simulink model "Last_Model_Interior_team"  (R2017b)
settings: Solver=VariableStepAuto  SolverName=FixedStepDiscrete  StartTime=0.0  StopTime=10  FixedStep=1e-6
PreLoadFcn:
  | %% Motor Parameters
  | Rs=6.9*10^-3;
  | Ld=220*10^-6;
  | Lq=265.4*10^-6;
  | Pm=87.78*10^-3;
  | P=4;
  | b=0.0019;
  | J=0.13;
  | f=50;
  | P_Rated=100000;
  | N_Rated=6320;
  | N_max=30000;
  | Tfl=P_Rated/(N_Rated*(2*pi/60));
  | Tl=0;
  | 
  | %% hardware impl
  | Vdc=340;
  | clocking=100;
  | fs=10000;
  | Ts=1/fs;
  | Irated=500;
  | Imax=500;
  | Id_MAX=-(Pm/Ld);
  | I_Limit=Irated;
  | I_fw=I_Limit;
  | Vmax=Vdc/sqrt(3);
  | update=2;
  | 
  | 
  | %% Inverter
  | Vdc=340;
  | deadtime=1e-6;
  | 
  | 
  | 
  | %% Tuning OF Id_Pole_Placment
  | zeta_Id=0.707;
  | Gamma_Id=0.9;
  | Wn_Id=(1/(1-Gamma_Id))*(Rs/Ld);
  | Kc_Id=(2*zeta_Id*Ld*Wn_Id)-Rs;
  | TAW_Id=((2*zeta_Id*Wn_Id*Ld)-Rs)/(Ld*Wn_Id*Wn_Id);
  | 
  | %% Tuning OF Iq_Pole_Placment
  | zeta_Iq=0.707;
  | Gamma_Iq=0.9;
  | Wn_Iq=(1/(1-Gamma_Iq))*(Rs/Lq);
  | Kc_Iq=(2*zeta_Iq*Lq*Wn_Iq)-Rs;
  | TAW_Iq=((2*zeta_Iq*Wn_Iq*Lq)-Rs)/(Lq*Wn_Iq*Wn_Iq);
  | 
  | 
  | 
  | %% Tuning of PI Using Symmetric Optimum For q phase
  | Tc=(1/fs)/update;
  | A=8;
  | Kp_SO_q=Lq/(A*(Tc)*1.5);
  | Ki_SO_q=1/((A^2)*1.5*Tc);
  | %% Tuning of PI Using Symmetric Optimum For d phase
  | Kp_SO_d=Ld/(A*(Tc)*1.5);
  | Ki_SO_d=1/((A^2)*1.5*Tc);
  | 
  | ... (+20 lines)
InitFcn:
  | %% Motor Parameters
  | Rs=6.9*10^-3;
  | Ld=220*10^-6;
  | Lq=265.4*10^-6;
  | Pm=87.78*10^-3;
  | P=4;
  | b=0.0019;
  | J=0.13;
  | f=50;
  | P_Rated=100000;
  | N_Rated=6320;
  | N_max=30000;
  | Tfl=P_Rated/(N_Rated*(2*pi/60));
  | Tl=0;
  | 
  | %% hardware impl
  | Vdc=340;
  | clocking=100;
  | fs=10000;
  | Ts=1/fs;
  | Irated=500;
  | Imax=500;
  | Id_MAX=-(Pm/Ld);
  | I_Limit=Irated;
  | I_fw=I_Limit;
  | Vmax=Vdc/sqrt(3);
  | update=2;
  | 
  | %% Inverter
  | Vdc=340;
  | deadtime=1e-6;
  | 
  | 
  | 
  | %% Tuning OF Id_Pole_Placment
  | zeta_Id=0.707;
  | Gamma_Id=0.9;
  | Wn_Id=(1/(1-Gamma_Id))*(Rs/Ld);
  | Kc_Id=(2*zeta_Id*Ld*Wn_Id)-Rs;
  | TAW_Id=((2*zeta_Id*Wn_Id*Ld)-Rs)/(Ld*Wn_Id*Wn_Id);
  | 
  | %% Tuning OF Iq_Pole_Placment
  | zeta_Iq=0.707;
  | Gamma_Iq=0.9;
  | Wn_Iq=(1/(1-Gamma_Iq))*(Rs/Lq);
  | Kc_Iq=(2*zeta_Iq*Lq*Wn_Iq)-Rs;
  | TAW_Iq=((2*zeta_Iq*Wn_Iq*Lq)-Rs)/(Lq*Wn_Iq*Wn_Iq);
  | 
  | 
  | 
  | %% Tuning of PI Using Symmetric Optimum For q phase
  | Tc=(1/fs)/update;
  | A=8;
  | Kp_SO_q=Lq/(A*(Tc)*1.5);
  | Ki_SO_q=1/((A^2)*1.5*Tc);
  | %% Tuning of PI Using Symmetric Optimum For d phase
  | Kp_SO_d=Ld/(A*(Tc)*1.5);
  | Ki_SO_d=1/((A^2)*1.5*Tc);
  | 
  | 
  | ... (+19 lines)
undefined symbols (not defined in the file): DiscIntNeverNeededParam, magnitude
libraries: simulink x81, powerlib x14
(part 2 of 4)

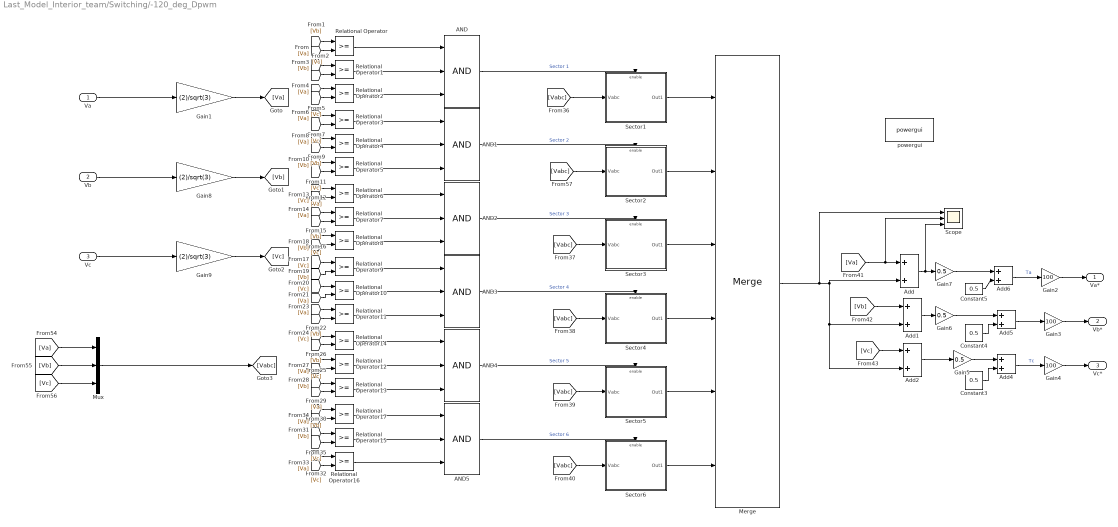
== system Last_Model_Interior_team/Switching/-120_deg_Dpwm ==
  Va : Inport
  Vb : Inport  Port=2
  Vc : Inport  Port=3
  AND{,1..5} (6 alike) : Logic  Inputs=3  IconShape=distinctive  AllPortsSameDT=off  OutDataTypeStr=boolean
  Add{,1..2,4..6} (6 alike) : Sum
  Constant3 : Constant  Value=0.5
  Constant4 : Constant  Value=0.5
  Constant5 : Constant  Value=0.5
  Gain1 : Gain  Gain=(2)/sqrt(3)  RndMeth=Simplest  OutDataTypeStr=Inherit: Same as input  ParamDataTypeStr=Inherit: Same as input
  Gain2 : Gain  Gain=100
  Gain3 : Gain  Gain=100
  Gain4 : Gain  Gain=100
  Gain5 : Gain  Gain=0.5
  Gain6 : Gain  Gain=0.5
  Gain7 : Gain  Gain=0.5
  Gain8 : Gain  Gain=(2)/sqrt(3)  RndMeth=Simplest  OutDataTypeStr=Inherit: Same as input  ParamDataTypeStr=Inherit: Same as input
  Gain9 : Gain  Gain=(2)/sqrt(3)  RndMeth=Simplest  OutDataTypeStr=Inherit: Same as input  ParamDataTypeStr=Inherit: Same as input
  Merge : Merge  Inputs=6
  Mux : Mux  Inputs=3
  Relational Operator{,1..17} (18 alike) : RelationalOperator  OutDataTypeStr=boolean  RndMeth=Simplest
  Scope : Scope  NumInputPorts=3
  Sector1 : Subsystem  TreatAsAtomicUnit=on
  Sector2 : Subsystem  TreatAsAtomicUnit=on
  Sector3 : Subsystem  TreatAsAtomicUnit=on
  Sector4 : Subsystem  TreatAsAtomicUnit=on
  Sector5 : Subsystem  TreatAsAtomicUnit=on
  Sector6 : Subsystem  TreatAsAtomicUnit=on
  powergui : powerlib/powergui  Priority=1  SimulationMode=Discrete  SampleTime=1e-6  frequency=60  Iterations=50  frequencyindice=0  Pbase=100e6  ErrMax=1e-4  UnitsV=kV  UnitsW=MW  buscounter=0  FunctionMessages=off  echomessages=off  EnableUseOfTLC=off  CurrentSourceSwitches=off  DisableSnubberDevices=off  DisableRonSwitches=off  DisableVfSwitches=off  DisplayEquations=off  AutomaticDiscreteSolvers=off  SolverType=Tustin/Backward Euler (TBE)  Interpol=off  ExternalGateDelay=off  methode=off  Ts=100  x0status=blocks  SPID=on  SwTol=0  HookPort=off  NonlinearTolerance=1e-4  nMaxIteration=100  ContinueOnMaxIteration=off  RestoreLinks=warning  ResistiveCurrentMeasurement=off  Frange=[0:2:500]  Ylog=off  Xlog=on  ShowGrid=off  save=off  variable=ZData  structure=0  ZoomFFT=off  StartTime=0.0  cycles=1  DisplayStyle=1  fundamental=60  FreqAxis=off  MaxFrequency=1000  frequencyindicesteady=1  RmsSteady=1  display=off
  Va* : Outport
  Vb* : Outport  Port=2
  Vc* : Outport  Port=3
  wires:
  AND5/1 -> Sector6/Enable  "Sector 6"
  AND4/1 -> Sector5/Enable  "Sector 5"
  AND3/1 -> Sector4/Enable  "Sector 4"
  AND2/1 -> Sector3/Enable  "Sector 3"
  AND1/1 -> Sector2/Enable  "Sector 2"
  AND/1 -> Sector1/Enable  "Sector 1"
  [Va] -> Relational Operator4/1
  [Va] -> Relational Operator2/1
  [Vb] -> Relational Operator11/2
  Relational Operator17/1 -> AND5/1
  [Va] -> Relational Operator12/2
  [Vabc] -> Sector4/1(Vabc)
  [Va] -> Relational Operator16/2
  [Vb] -> Relational Operator13/1
  [Vc] -> Relational Operator5/2
  [Vb] -> Relational Operator/1
  [Vabc] -> Sector5/1(Vabc)
  [Va] -> Scope/2, Add/1
  Relational Operator11/1 -> AND3/3
  [Vb] -> Relational Operator15/1
  [Vc] -> Relational Operator2/2
  Relational Operator16/1 -> AND5/3
  [Va] -> Relational Operator17/2
  Relational Operator15/1 -> AND5/2
  Relational Operator12/1 -> AND4/2
  [Va] -> Relational Operator3/1
  [Va] -> Relational Operator/2
  Relational Operator/1 -> AND/1
  Relational Operator3/1 -> AND1/1
  [Vc] -> Mux/3
  Sector1/1(Out1) -> Merge/1
  Gain4/1 -> Vc*/1
  [Vb] -> Relational Operator1/1
  [Vb] -> Relational Operator4/2
  Gain6/1 -> Add5/1
  [Vb] -> Relational Operator17/1
  Gain2/1 -> Va*/1
  Relational Operator1/1 -> AND/2
  Relational Operator9/1 -> AND3/1
  [Va] -> Relational Operator11/1
  [Va] -> Mux/1
  [Vc] -> Relational Operator12/1
  Relational Operator7/1 -> AND2/2
  [Vabc] -> Sector6/1(Vabc)
  [Vc] -> Relational Operator15/2
  Relational Operator2/1 -> AND/3
  [Vc] -> Relational Operator3/2
  [Vb] -> Mux/2
  [Vc] -> Relational Operator14/1
  [Vc] -> Relational Operator10/1
  Relational Operator13/1 -> AND4/3
  Relational Operator14/1 -> AND4/1
  [Vc] -> Relational Operator9/1
  [Vabc] -> Sector1/1(Vabc)
  Relational Operator10/1 -> AND3/2
  Add1/1 -> Gain6/1
  [Vb] -> Relational Operator5/1
  Relational Operator5/1 -> AND1/3
  Relational Operator4/1 -> AND1/2
  Relational Operator6/1 -> AND2/1
  Relational Operator8/1 -> AND2/3
  [Vc] -> Relational Operator1/2
  [Vc] -> Relational Operator8/1
  [Vabc] -> Sector2/1(Vabc)
  [Vc] -> Relational Operator16/1
  [Vb] -> Relational Operator14/2
  [Vb] -> Relational Operator9/2
  [Vb] -> Relational Operator7/2
  [Vc] -> Relational Operator6/2
  [Va] -> Relational Operator6/1
  Gain3/1 -> Vb*/1
  [Va] -> Relational Operator7/1
  [Va] -> Relational Operator13/2
  [Vb] -> Relational Operator8/2
  [Va] -> Relational Operator10/2
  Sector2/1(Out1) -> Merge/2
  Sector6/1(Out1) -> Merge/6
  [Vabc] -> Sector3/1(Vabc)
  Sector3/1(Out1) -> Merge/3
  Sector5/1(Out1) -> Merge/5
  Sector4/1(Out1) -> Merge/4
  [Vc] -> Add2/1
  [Vb] -> Add1/1
  Gain5/1 -> Add4/1
  Constant3/1 -> Add4/2
  Constant4/1 -> Add5/2
  Gain7/1 -> Add6/1
  Constant5/1 -> Add6/2
  Add2/1 -> Gain5/1
  Add5/1 -> Gain3/1
  Add4/1 -> Gain4/1  "Tc"
  Add6/1 -> Gain2/1  "Ta"
  Mux/1 -> [Vabc]
  Vc/1 -> Gain9/1
  Vb/1 -> Gain8/1
  Va/1 -> Gain1/1
  Merge/1 -> Scope/1, Add/2, Add2/2, Add1/2
  Add/1 -> Scope/3, Gain7/1
  Gain1/1 -> [Va]
  Gain8/1 -> [Vb]
  Gain9/1 -> [Vc]

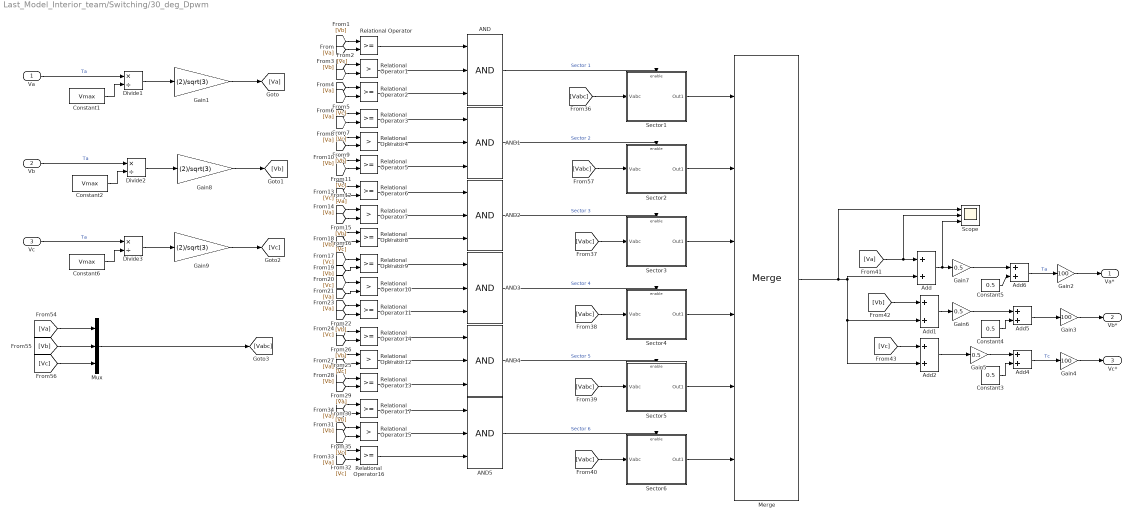
== system Last_Model_Interior_team/Switching/30_deg_Dpwm ==
  Va : Inport
  Vb : Inport  Port=2
  Vc : Inport  Port=3
  AND{,1..5} (6 alike) : Logic  Inputs=3  IconShape=distinctive  AllPortsSameDT=off  OutDataTypeStr=boolean
  Add{,1..2,4..6} (6 alike) : Sum
  Constant1 : Constant  Value=Vmax
  Constant2 : Constant  Value=Vmax
  Constant3 : Constant  Value=0.5
  Constant4 : Constant  Value=0.5
  Constant5 : Constant  Value=0.5
  Constant6 : Constant  Value=Vmax
  Divide1 : Product  Inputs=*/
  Divide2 : Product  Inputs=*/
  Divide3 : Product  Inputs=*/
  Gain1 : Gain  Gain=(2)/sqrt(3)  RndMeth=Simplest  OutDataTypeStr=Inherit: Same as input  ParamDataTypeStr=Inherit: Same as input
  Gain2 : Gain  Gain=100
  Gain3 : Gain  Gain=100
  Gain4 : Gain  Gain=100
  Gain5 : Gain  Gain=0.5
  Gain6 : Gain  Gain=0.5
  Gain7 : Gain  Gain=0.5
  Gain8 : Gain  Gain=(2)/sqrt(3)  RndMeth=Simplest  OutDataTypeStr=Inherit: Same as input  ParamDataTypeStr=Inherit: Same as input
  Gain9 : Gain  Gain=(2)/sqrt(3)  RndMeth=Simplest  OutDataTypeStr=Inherit: Same as input  ParamDataTypeStr=Inherit: Same as input
  Merge : Merge  Inputs=6
  Mux : Mux  Inputs=3
  Relational Operator{,2..3,5..6,8..9,11,13..14,16..17} (12 alike) : RelationalOperator  OutDataTypeStr=boolean  RndMeth=Simplest
  Relational Operator{1,4,7,10,12,15} (6 alike) : RelationalOperator  Operator=>  OutDataTypeStr=boolean  RndMeth=Simplest
  Scope : Scope  NumInputPorts=3
  Sector1 : Subsystem  TreatAsAtomicUnit=on
  Sector2 : Subsystem  TreatAsAtomicUnit=on
  Sector3 : Subsystem  TreatAsAtomicUnit=on
  Sector4 : Subsystem  TreatAsAtomicUnit=on
  Sector5 : Subsystem  TreatAsAtomicUnit=on
  Sector6 : Subsystem  TreatAsAtomicUnit=on
  Va* : Outport
  Vb* : Outport  Port=2
  Vc* : Outport  Port=3
  wires:
  Add/1 -> Gain7/1, Scope/3
  Merge/1 -> Add1/2, Add2/2, Add/2, Scope/1
  Add6/1 -> Gain2/1  "Ta"
  Add4/1 -> Gain4/1  "Tc"
  Add5/1 -> Gain3/1
  Add2/1 -> Gain5/1
  Constant5/1 -> Add6/2
  Gain7/1 -> Add6/1
  Constant4/1 -> Add5/2
  Constant3/1 -> Add4/2
  Gain5/1 -> Add4/1
  [Vb] -> Add1/1
  [Vc] -> Add2/1
  Sector4/1(Out1) -> Merge/4
  Sector5/1(Out1) -> Merge/5
  Sector3/1(Out1) -> Merge/3
  [Vabc] -> Sector3/1(Vabc)
  Sector6/1(Out1) -> Merge/6
  Sector2/1(Out1) -> Merge/2
  [Va] -> Relational Operator10/2
  [Vb] -> Relational Operator8/2
  [Va] -> Relational Operator13/2
  [Va] -> Relational Operator7/1
  Gain3/1 -> Vb*/1
  [Va] -> Relational Operator6/1
  [Vc] -> Relational Operator6/2
  [Vb] -> Relational Operator7/2
  [Vb] -> Relational Operator9/2
  [Vb] -> Relational Operator14/2
  [Vc] -> Relational Operator16/1
  [Vabc] -> Sector2/1(Vabc)
  [Vc] -> Relational Operator8/1
  [Vc] -> Relational Operator1/2
  Relational Operator8/1 -> AND2/3
  Relational Operator6/1 -> AND2/1
  Relational Operator4/1 -> AND1/2
  Relational Operator5/1 -> AND1/3
  [Vb] -> Relational Operator5/1
  Add1/1 -> Gain6/1
  Relational Operator10/1 -> AND3/2
  [Vabc] -> Sector1/1(Vabc)
  [Vc] -> Relational Operator9/1
  Relational Operator14/1 -> AND4/1
  Relational Operator13/1 -> AND4/3
  [Vc] -> Relational Operator10/1
  [Vc] -> Relational Operator14/1
  [Vc] -> Relational Operator3/2
  Relational Operator2/1 -> AND/3
  [Vc] -> Relational Operator15/2
  [Vabc] -> Sector6/1(Vabc)
  Relational Operator7/1 -> AND2/2
  [Vc] -> Relational Operator12/1
  [Va] -> Relational Operator11/1
  Relational Operator9/1 -> AND3/1
  Relational Operator1/1 -> AND/2
  Gain2/1 -> Va*/1
  [Vb] -> Relational Operator17/1
  Gain6/1 -> Add5/1
  [Vb] -> Relational Operator4/2
  [Vb] -> Relational Operator1/1
  Gain4/1 -> Vc*/1
  Sector1/1(Out1) -> Merge/1
  Relational Operator3/1 -> AND1/1
  Relational Operator/1 -> AND/1
  [Va] -> Relational Operator/2
  [Va] -> Relational Operator3/1
  Relational Operator12/1 -> AND4/2
  Relational Operator15/1 -> AND5/2
  [Va] -> Relational Operator17/2
  Relational Operator16/1 -> AND5/3
  [Vc] -> Relational Operator2/2
  [Vb] -> Relational Operator15/1
  Relational Operator11/1 -> AND3/3
  [Va] -> Add/1, Scope/2
  [Vabc] -> Sector5/1(Vabc)
  [Vb] -> Relational Operator/1
  [Vc] -> Relational Operator5/2
  [Vb] -> Relational Operator13/1
  [Va] -> Relational Operator16/2
  [Vabc] -> Sector4/1(Vabc)
  [Va] -> Relational Operator12/2
  Relational Operator17/1 -> AND5/1
  [Vb] -> Relational Operator11/2
  [Va] -> Relational Operator2/1
  [Va] -> Relational Operator4/1
  AND/1 -> Sector1/Enable  "Sector 1"
  AND1/1 -> Sector2/Enable  "Sector 2"
  AND2/1 -> Sector3/Enable  "Sector 3"
  AND3/1 -> Sector4/Enable  "Sector 4"
  AND4/1 -> Sector5/Enable  "Sector 5"
  AND5/1 -> Sector6/Enable  "Sector 6"
  Constant1/1 -> Divide1/2
  Vb/1 -> Divide2/1  "Ta"
  Divide1/1 -> Gain1/1
  Constant6/1 -> Divide3/2
  Divide3/1 -> Gain9/1
  Vc/1 -> Divide3/1  "Ta"
  Constant2/1 -> Divide2/2
  Divide2/1 -> Gain8/1
  Mux/1 -> [Vabc]
  [Vb] -> Mux/2
  Gain1/1 -> [Va]
  [Vc] -> Mux/3
  [Va] -> Mux/1
  Gain8/1 -> [Vb]
  Gain9/1 -> [Vc]
  Va/1 -> Divide1/1  "Ta"

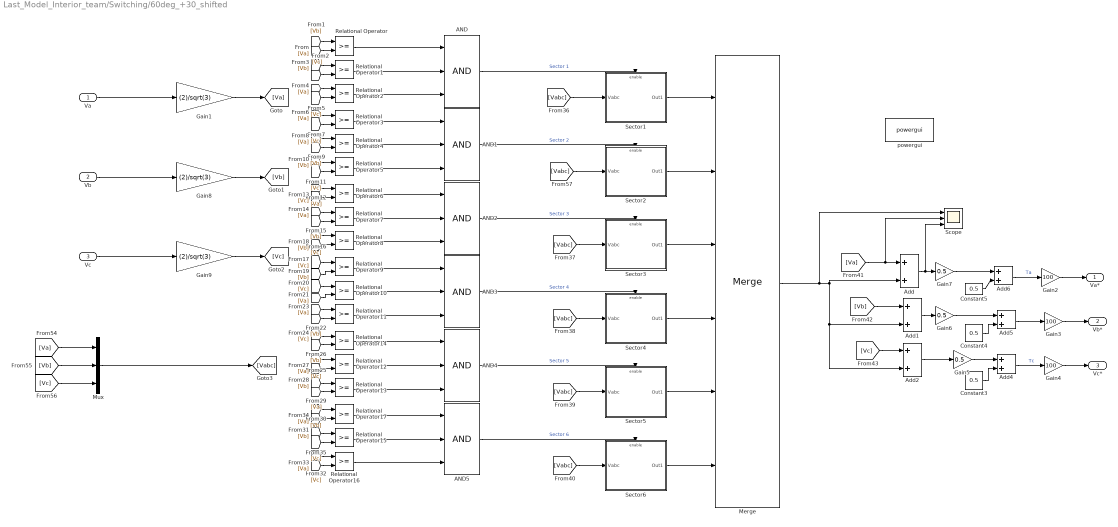
== system Last_Model_Interior_team/Switching/60deg_+30_shifted ==
  Va : Inport
  Vb : Inport  Port=2
  Vc : Inport  Port=3
  AND{,1..5} (6 alike) : Logic  Inputs=3  IconShape=distinctive  AllPortsSameDT=off  OutDataTypeStr=boolean
  Add{,1..2,4..6} (6 alike) : Sum
  Constant3 : Constant  Value=0.5
  Constant4 : Constant  Value=0.5
  Constant5 : Constant  Value=0.5
  Gain1 : Gain  Gain=(2)/sqrt(3)  RndMeth=Simplest  OutDataTypeStr=Inherit: Same as input  ParamDataTypeStr=Inherit: Same as input
  Gain2 : Gain  Gain=100
  Gain3 : Gain  Gain=100
  Gain4 : Gain  Gain=100
  Gain5 : Gain  Gain=0.5
  Gain6 : Gain  Gain=0.5
  Gain7 : Gain  Gain=0.5
  Gain8 : Gain  Gain=(2)/sqrt(3)  RndMeth=Simplest  OutDataTypeStr=Inherit: Same as input  ParamDataTypeStr=Inherit: Same as input
  Gain9 : Gain  Gain=(2)/sqrt(3)  RndMeth=Simplest  OutDataTypeStr=Inherit: Same as input  ParamDataTypeStr=Inherit: Same as input
  Merge : Merge  Inputs=6
  Mux : Mux  Inputs=3
  Relational Operator{,1..17} (18 alike) : RelationalOperator  OutDataTypeStr=boolean  RndMeth=Simplest
  Scope : Scope  NumInputPorts=3
  Sector1 : Subsystem  TreatAsAtomicUnit=on
  Sector2 : Subsystem  TreatAsAtomicUnit=on
  Sector3 : Subsystem  TreatAsAtomicUnit=on
  Sector4 : Subsystem  TreatAsAtomicUnit=on
  Sector5 : Subsystem  TreatAsAtomicUnit=on
  Sector6 : Subsystem  TreatAsAtomicUnit=on
  powergui : powerlib/powergui  Priority=1  SimulationMode=Discrete  SampleTime=1e-6  frequency=60  Iterations=50  frequencyindice=0  Pbase=100e6  ErrMax=1e-4  UnitsV=kV  UnitsW=MW  buscounter=0  FunctionMessages=off  echomessages=off  EnableUseOfTLC=off  CurrentSourceSwitches=off  DisableSnubberDevices=off  DisableRonSwitches=off  DisableVfSwitches=off  DisplayEquations=off  AutomaticDiscreteSolvers=off  SolverType=Tustin/Backward Euler (TBE)  Interpol=off  ExternalGateDelay=off  methode=off  Ts=100  x0status=blocks  SPID=on  SwTol=0  HookPort=off  NonlinearTolerance=1e-4  nMaxIteration=100  ContinueOnMaxIteration=off  RestoreLinks=warning  ResistiveCurrentMeasurement=off  Frange=[0:2:500]  Ylog=off  Xlog=on  ShowGrid=off  save=off  variable=ZData  structure=0  ZoomFFT=off  StartTime=0.0  cycles=1  DisplayStyle=1  fundamental=60  FreqAxis=off  MaxFrequency=1000  frequencyindicesteady=1  RmsSteady=1  display=off
  Va* : Outport
  Vb* : Outport  Port=2
  Vc* : Outport  Port=3
  wires:
  [Va] -> Relational Operator4/1
  [Va] -> Relational Operator2/1
  [Vb] -> Relational Operator11/2
  AND5/1 -> Sector6/Enable  "Sector 6"
  Relational Operator17/1 -> AND5/1
  [Va] -> Relational Operator12/2
  [Vabc] -> Sector4/1(Vabc)
  [Va] -> Relational Operator16/2
  AND3/1 -> Sector4/Enable  "Sector 4"
  AND/1 -> Sector1/Enable  "Sector 1"
  [Vb] -> Relational Operator13/1
  [Vc] -> Relational Operator5/2
  [Vb] -> Relational Operator/1
  [Vabc] -> Sector5/1(Vabc)
  [Va] -> Scope/2, Add/1
  Relational Operator11/1 -> AND3/3
  [Vb] -> Relational Operator15/1
  [Vc] -> Relational Operator2/2
  Relational Operator16/1 -> AND5/3
  [Va] -> Relational Operator17/2
  Relational Operator15/1 -> AND5/2
  Relational Operator12/1 -> AND4/2
  [Va] -> Relational Operator3/1
  [Va] -> Relational Operator/2
  Relational Operator/1 -> AND/1
  AND4/1 -> Sector5/Enable  "Sector 5"
  Relational Operator3/1 -> AND1/1
  [Vc] -> Mux/3
  Sector1/1(Out1) -> Merge/1
  Gain4/1 -> Vc*/1
  [Vb] -> Relational Operator1/1
  [Vb] -> Relational Operator4/2
  Gain6/1 -> Add5/1
  [Vb] -> Relational Operator17/1
  Gain2/1 -> Va*/1
  Relational Operator1/1 -> AND/2
  Relational Operator9/1 -> AND3/1
  [Va] -> Relational Operator11/1
  [Va] -> Mux/1
  [Vc] -> Relational Operator12/1
  AND2/1 -> Sector3/Enable  "Sector 3"
  Relational Operator7/1 -> AND2/2
  [Vabc] -> Sector6/1(Vabc)
  [Vc] -> Relational Operator15/2
  Relational Operator2/1 -> AND/3
  [Vc] -> Relational Operator3/2
  [Vb] -> Mux/2
  [Vc] -> Relational Operator14/1
  [Vc] -> Relational Operator10/1
  Relational Operator13/1 -> AND4/3
  Relational Operator14/1 -> AND4/1
  [Vc] -> Relational Operator9/1
  [Vabc] -> Sector1/1(Vabc)
  Relational Operator10/1 -> AND3/2
  Add1/1 -> Gain6/1
  [Vb] -> Relational Operator5/1
  Relational Operator5/1 -> AND1/3
  Relational Operator4/1 -> AND1/2
  Relational Operator6/1 -> AND2/1
  Relational Operator8/1 -> AND2/3
  [Vc] -> Relational Operator1/2
  [Vc] -> Relational Operator8/1
  [Vabc] -> Sector2/1(Vabc)
  [Vc] -> Relational Operator16/1
  [Vb] -> Relational Operator14/2
  [Vb] -> Relational Operator9/2
  [Vb] -> Relational Operator7/2
  [Vc] -> Relational Operator6/2
  [Va] -> Relational Operator6/1
  Gain3/1 -> Vb*/1
  [Va] -> Relational Operator7/1
  [Va] -> Relational Operator13/2
  [Vb] -> Relational Operator8/2
  [Va] -> Relational Operator10/2
  Sector2/1(Out1) -> Merge/2
  Sector6/1(Out1) -> Merge/6
  [Vabc] -> Sector3/1(Vabc)
  Sector3/1(Out1) -> Merge/3
  AND1/1 -> Sector2/Enable  "Sector 2"
  Sector5/1(Out1) -> Merge/5
  Sector4/1(Out1) -> Merge/4
  [Vc] -> Add2/1
  [Vb] -> Add1/1
  Gain5/1 -> Add4/1
  Constant3/1 -> Add4/2
  Constant4/1 -> Add5/2
  Gain7/1 -> Add6/1
  Constant5/1 -> Add6/2
  Add2/1 -> Gain5/1
  Add5/1 -> Gain3/1
  Add4/1 -> Gain4/1  "Tc"
  Add6/1 -> Gain2/1  "Ta"
  Mux/1 -> [Vabc]
  Vc/1 -> Gain9/1
  Vb/1 -> Gain8/1
  Va/1 -> Gain1/1
  Merge/1 -> Scope/1, Add/2, Add2/2, Add1/2
  Add/1 -> Scope/3, Gain7/1
  Gain1/1 -> [Va]
  Gain8/1 -> [Vb]
  Gain9/1 -> [Vc]

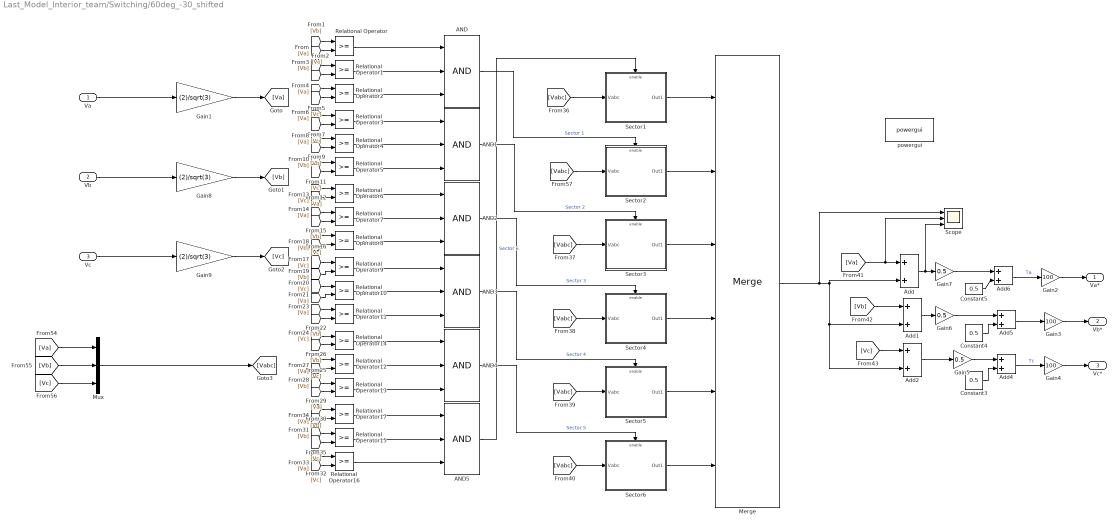
== system Last_Model_Interior_team/Switching/60deg_-30_shifted ==
  Va : Inport
  Vb : Inport  Port=2
  Vc : Inport  Port=3
  AND{,1..5} (6 alike) : Logic  Inputs=3  IconShape=distinctive  AllPortsSameDT=off  OutDataTypeStr=boolean
  Add{,1..2,4..6} (6 alike) : Sum
  Constant3 : Constant  Value=0.5
  Constant4 : Constant  Value=0.5
  Constant5 : Constant  Value=0.5
  Gain1 : Gain  Gain=(2)/sqrt(3)  RndMeth=Simplest  OutDataTypeStr=Inherit: Same as input  ParamDataTypeStr=Inherit: Same as input
  Gain2 : Gain  Gain=100
  Gain3 : Gain  Gain=100
  Gain4 : Gain  Gain=100
  Gain5 : Gain  Gain=0.5
  Gain6 : Gain  Gain=0.5
  Gain7 : Gain  Gain=0.5
  Gain8 : Gain  Gain=(2)/sqrt(3)  RndMeth=Simplest  OutDataTypeStr=Inherit: Same as input  ParamDataTypeStr=Inherit: Same as input
  Gain9 : Gain  Gain=(2)/sqrt(3)  RndMeth=Simplest  OutDataTypeStr=Inherit: Same as input  ParamDataTypeStr=Inherit: Same as input
  Merge : Merge  Inputs=6
  Mux : Mux  Inputs=3
  Relational Operator{,1..17} (18 alike) : RelationalOperator  OutDataTypeStr=boolean  RndMeth=Simplest
  Scope : Scope  NumInputPorts=3
  Sector1 : Subsystem  TreatAsAtomicUnit=on
  Sector2 : Subsystem  TreatAsAtomicUnit=on
  Sector3 : Subsystem  TreatAsAtomicUnit=on
  Sector4 : Subsystem  TreatAsAtomicUnit=on
  Sector5 : Subsystem  TreatAsAtomicUnit=on
  Sector6 : Subsystem  TreatAsAtomicUnit=on
  powergui : powerlib/powergui  Priority=1  SimulationMode=Discrete  SampleTime=1e-6  frequency=60  Iterations=50  frequencyindice=0  Pbase=100e6  ErrMax=1e-4  UnitsV=kV  UnitsW=MW  buscounter=0  FunctionMessages=off  echomessages=off  EnableUseOfTLC=off  CurrentSourceSwitches=off  DisableSnubberDevices=off  DisableRonSwitches=off  DisableVfSwitches=off  DisplayEquations=off  AutomaticDiscreteSolvers=off  SolverType=Tustin/Backward Euler (TBE)  Interpol=off  ExternalGateDelay=off  methode=off  Ts=100  x0status=blocks  SPID=on  SwTol=0  HookPort=off  NonlinearTolerance=1e-4  nMaxIteration=100  ContinueOnMaxIteration=off  RestoreLinks=warning  ResistiveCurrentMeasurement=off  Frange=[0:2:500]  Ylog=off  Xlog=on  ShowGrid=off  save=off  variable=ZData  structure=0  ZoomFFT=off  StartTime=0.0  cycles=1  DisplayStyle=1  fundamental=60  FreqAxis=off  MaxFrequency=1000  frequencyindicesteady=1  RmsSteady=1  display=off
  Va* : Outport
  Vb* : Outport  Port=2
  Vc* : Outport  Port=3
  wires:
  Gain9/1 -> [Vc]
  Gain8/1 -> [Vb]
  Gain1/1 -> [Va]
  Add/1 -> Gain7/1, Scope/3
  Merge/1 -> Add1/2, Add2/2, Add/2, Scope/1
  Va/1 -> Gain1/1
  Vb/1 -> Gain8/1
  Vc/1 -> Gain9/1
  Mux/1 -> [Vabc]
  Add6/1 -> Gain2/1  "Ta"
  Add4/1 -> Gain4/1  "Tc"
  Add5/1 -> Gain3/1
  Add2/1 -> Gain5/1
  Constant5/1 -> Add6/2
  Gain7/1 -> Add6/1
  Constant4/1 -> Add5/2
  Constant3/1 -> Add4/2
  Gain5/1 -> Add4/1
  [Vb] -> Add1/1
  [Vc] -> Add2/1
  Sector4/1(Out1) -> Merge/4
  Sector5/1(Out1) -> Merge/5
  Sector3/1(Out1) -> Merge/3
  [Vabc] -> Sector3/1(Vabc)
  Sector6/1(Out1) -> Merge/6
  Sector2/1(Out1) -> Merge/2
  [Va] -> Relational Operator10/2
  [Vb] -> Relational Operator8/2
  [Va] -> Relational Operator13/2
  [Va] -> Relational Operator7/1
  Gain3/1 -> Vb*/1
  [Va] -> Relational Operator6/1
  [Vc] -> Relational Operator6/2
  [Vb] -> Relational Operator7/2
  [Vb] -> Relational Operator9/2
  [Vb] -> Relational Operator14/2
  [Vc] -> Relational Operator16/1
  [Vabc] -> Sector2/1(Vabc)
  [Vc] -> Relational Operator8/1
  [Vc] -> Relational Operator1/2
  Relational Operator8/1 -> AND2/3
  Relational Operator6/1 -> AND2/1
  Relational Operator4/1 -> AND1/2
  Relational Operator5/1 -> AND1/3
  [Vb] -> Relational Operator5/1
  Add1/1 -> Gain6/1
  Relational Operator10/1 -> AND3/2
  [Vabc] -> Sector1/1(Vabc)
  [Vc] -> Relational Operator9/1
  Relational Operator14/1 -> AND4/1
  Relational Operator13/1 -> AND4/3
  [Vc] -> Relational Operator10/1
  [Vc] -> Relational Operator14/1
  [Vb] -> Mux/2
  [Vc] -> Relational Operator3/2
  Relational Operator2/1 -> AND/3
  [Vc] -> Relational Operator15/2
  [Vabc] -> Sector6/1(Vabc)
  Relational Operator7/1 -> AND2/2
  [Vc] -> Relational Operator12/1
  [Va] -> Mux/1
  [Va] -> Relational Operator11/1
  Relational Operator9/1 -> AND3/1
  Relational Operator1/1 -> AND/2
  Gain2/1 -> Va*/1
  [Vb] -> Relational Operator17/1
  Gain6/1 -> Add5/1
  [Vb] -> Relational Operator4/2
  [Vb] -> Relational Operator1/1
  Gain4/1 -> Vc*/1
  Sector1/1(Out1) -> Merge/1
  [Vc] -> Mux/3
  Relational Operator3/1 -> AND1/1
  Relational Operator/1 -> AND/1
  [Va] -> Relational Operator/2
  [Va] -> Relational Operator3/1
  Relational Operator12/1 -> AND4/2
  Relational Operator15/1 -> AND5/2
  [Va] -> Relational Operator17/2
  Relational Operator16/1 -> AND5/3
  [Vc] -> Relational Operator2/2
  [Vb] -> Relational Operator15/1
  Relational Operator11/1 -> AND3/3
  [Va] -> Add/1, Scope/2
  [Vabc] -> Sector5/1(Vabc)
  [Vb] -> Relational Operator/1
  [Vc] -> Relational Operator5/2
  [Vb] -> Relational Operator13/1
  [Va] -> Relational Operator16/2
  [Vabc] -> Sector4/1(Vabc)
  [Va] -> Relational Operator12/2
  Relational Operator17/1 -> AND5/1
  [Vb] -> Relational Operator11/2
  [Va] -> Relational Operator2/1
  [Va] -> Relational Operator4/1
  AND1/1 -> Sector3/Enable  "Sector 2"
  AND2/1 -> Sector4/Enable  "Sector 3"
  AND/1 -> Sector2/Enable  "Sector 1"
  AND3/1 -> Sector5/Enable  "Sector 4"
  AND4/1 -> Sector6/Enable  "Sector 5"
  AND5/1 -> Sector1/Enable  "Sector 6"

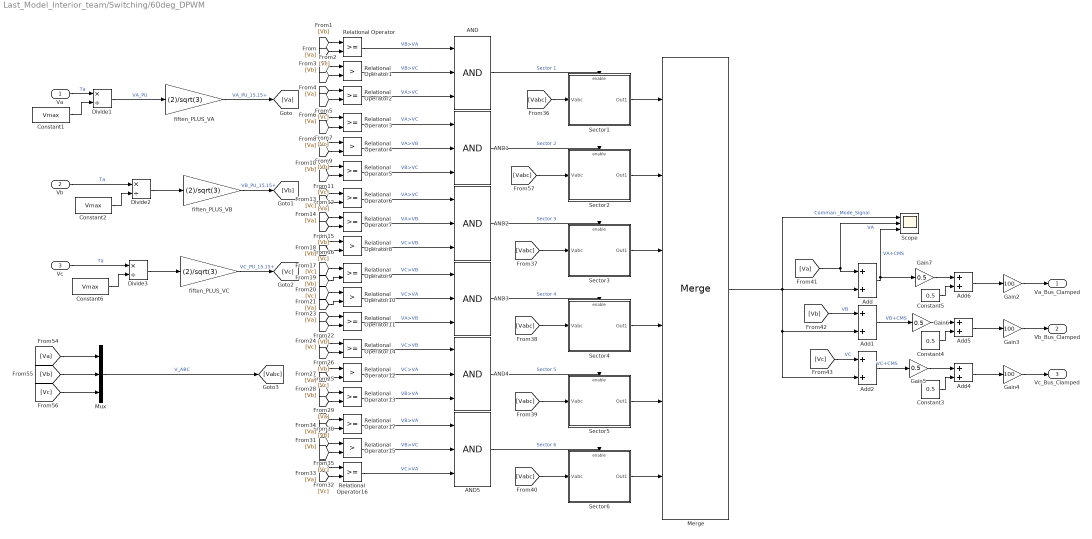
== system Last_Model_Interior_team/Switching/60deg_DPWM ==
  Va : Inport
  Vb : Inport  Port=2
  Vc : Inport  Port=3
  AND{,1..5} (6 alike) : Logic  Inputs=3  IconShape=distinctive  AllPortsSameDT=off  OutDataTypeStr=boolean
  Add{,1..2,4..6} (6 alike) : Sum
  Constant1 : Constant  Value=Vmax
  Constant2 : Constant  Value=Vmax
  Constant3 : Constant  Value=0.5
  Constant4 : Constant  Value=0.5
  Constant5 : Constant  Value=0.5
  Constant6 : Constant  Value=Vmax
  Divide1 : Product  Inputs=*/
  Divide2 : Product  Inputs=*/
  Divide3 : Product  Inputs=*/
  Gain2 : Gain  Gain=100
  Gain3 : Gain  Gain=100
  Gain4 : Gain  Gain=100
  Gain5 : Gain  Gain=0.5
  Gain6 : Gain  Gain=0.5
  Gain7 : Gain  Gain=0.5
  Merge : Merge  Inputs=6
  Mux : Mux  Inputs=3
  Relational Operator{,2..3,5..7,9,11,13..14,16..17} (12 alike) : RelationalOperator  OutDataTypeStr=boolean  RndMeth=Simplest
  Relational Operator{1,4,8,10,12,15} (6 alike) : RelationalOperator  Operator=>  OutDataTypeStr=boolean  RndMeth=Simplest
  Scope : Scope  NumInputPorts=3
  Sector1 : Subsystem  TreatAsAtomicUnit=on
  Sector2 : Subsystem  TreatAsAtomicUnit=on
  Sector3 : Subsystem  TreatAsAtomicUnit=on
  Sector4 : Subsystem  TreatAsAtomicUnit=on
  Sector5 : Subsystem  TreatAsAtomicUnit=on
  Sector6 : Subsystem  TreatAsAtomicUnit=on
  fiften_PLUS_VA : Gain  Gain=(2)/sqrt(3)  RndMeth=Simplest  OutDataTypeStr=Inherit: Same as input  ParamDataTypeStr=Inherit: Same as input
  fiften_PLUS_VB : Gain  Gain=(2)/sqrt(3)  RndMeth=Simplest  OutDataTypeStr=Inherit: Same as input  ParamDataTypeStr=Inherit: Same as input
  fiften_PLUS_VC : Gain  Gain=(2)/sqrt(3)  RndMeth=Simplest  OutDataTypeStr=Inherit: Same as input  ParamDataTypeStr=Inherit: Same as input
  Va_Bus_Clamped : Outport
  Vb_Bus_Clamped : Outport  Port=2
  Vc_Bus_Clamped : Outport  Port=3
  wires:
  [Va] -> Relational Operator4/1
  [Va] -> Relational Operator2/1
  [Vb] -> Relational Operator11/2
  AND5/1 -> Sector6/Enable  "Sector 6"
  Relational Operator17/1 -> AND5/1  "VB>VA"
  [Va] -> Relational Operator12/2
  [Vabc] -> Sector4/1(Vabc)
  [Va] -> Relational Operator16/2
  AND3/1 -> Sector4/Enable  "Sector 4"
  AND/1 -> Sector1/Enable  "Sector 1"
  [Vb] -> Relational Operator13/1
  [Vc] -> Relational Operator5/2
  [Vb] -> Relational Operator/1
  [Vabc] -> Sector5/1(Vabc)
  [Va] -> Scope/2, Add/1  "VA"
  Relational Operator11/1 -> AND3/3  "VA>VB"
  [Vb] -> Relational Operator15/1
  [Vc] -> Relational Operator2/2
  Relational Operator16/1 -> AND5/3  "VC>VA"
  [Va] -> Relational Operator17/2
  Relational Operator15/1 -> AND5/2  "VB>VC"
  Relational Operator12/1 -> AND4/2  "VC>VA"
  [Va] -> Relational Operator3/1
  [Va] -> Relational Operator/2
  Relational Operator/1 -> AND/1  "VB>VA"
  AND4/1 -> Sector5/Enable  "Sector 5"
  Relational Operator3/1 -> AND1/1  "VA>VC"
  [Vc] -> Mux/3
  Sector1/1(Out1) -> Merge/1
  Gain4/1 -> Vc_Bus_Clamped/1
  [Vb] -> Relational Operator1/1
  [Vb] -> Relational Operator4/2
  Gain6/1 -> Add5/1
  [Vb] -> Relational Operator17/1
  Gain2/1 -> Va_Bus_Clamped/1
  Relational Operator1/1 -> AND/2  "VB>VC"
  Relational Operator9/1 -> AND3/1  "VC>VB"
  [Va] -> Relational Operator11/1
  [Va] -> Mux/1
  [Vc] -> Relational Operator12/1
  AND2/1 -> Sector3/Enable  "Sector 3"
  Relational Operator7/1 -> AND2/2  "VA>VB"
  [Vabc] -> Sector6/1(Vabc)
  [Vc] -> Relational Operator15/2
  Relational Operator2/1 -> AND/3  "VA>VC"
  [Vc] -> Relational Operator3/2
  [Vb] -> Mux/2
  [Vc] -> Relational Operator14/1
  [Vc] -> Relational Operator10/1
  Relational Operator13/1 -> AND4/3  "VB>VA"
  Relational Operator14/1 -> AND4/1  "VC>VB"
  [Vc] -> Relational Operator9/1
  [Vabc] -> Sector1/1(Vabc)
  Relational Operator10/1 -> AND3/2  "VC>VA"
  Add1/1 -> Gain6/1  "VB+CMS"
  [Vb] -> Relational Operator5/1
  Relational Operator5/1 -> AND1/3  "VB>VC"
  Relational Operator4/1 -> AND1/2  "VA>VB"
  Relational Operator6/1 -> AND2/1  "VA>VC"
  Relational Operator8/1 -> AND2/3  "VC>VB"
  [Vc] -> Relational Operator1/2
  [Vc] -> Relational Operator8/1
  [Vabc] -> Sector2/1(Vabc)
  [Vc] -> Relational Operator16/1
  [Vb] -> Relational Operator14/2
  [Vb] -> Relational Operator9/2
  [Vb] -> Relational Operator7/2
  [Vc] -> Relational Operator6/2
  [Va] -> Relational Operator6/1
  Gain3/1 -> Vb_Bus_Clamped/1
  [Va] -> Relational Operator7/1
  [Va] -> Relational Operator13/2
  [Vb] -> Relational Operator8/2
  [Va] -> Relational Operator10/2
  Sector2/1(Out1) -> Merge/2
  Sector6/1(Out1) -> Merge/6
  [Vabc] -> Sector3/1(Vabc)
  Sector3/1(Out1) -> Merge/3
  AND1/1 -> Sector2/Enable  "Sector 2"
  Sector5/1(Out1) -> Merge/5
  Sector4/1(Out1) -> Merge/4
  [Vc] -> Add2/1  "VC"
  [Vb] -> Add1/1  "VB"
  Gain5/1 -> Add4/1
  Constant3/1 -> Add4/2
  Constant4/1 -> Add5/2
  Gain7/1 -> Add6/1
  Constant5/1 -> Add6/2
  Add2/1 -> Gain5/1  "VC+CMS"
  Add5/1 -> Gain3/1
  Add4/1 -> Gain4/1
  Add6/1 -> Gain2/1
  Mux/1 -> [Vabc]  "V_ABC"
  Merge/1 -> Scope/1, Add/2, Add2/2, Add1/2  "Comman _Mode_Signal"
  Add/1 -> Scope/3, Gain7/1  "VA+CMS"
  fiften_PLUS_VA/1 -> [Va]  "VA_PU_15.15+"
  fiften_PLUS_VB/1 -> [Vb]  "VB_PU_15.15+"
  fiften_PLUS_VC/1 -> [Vc]  "VC_PU_15.15+"
  Va/1 -> Divide1/1  "Ta"
  Constant1/1 -> Divide1/2
  Divide1/1 -> fiften_PLUS_VA/1  "VA_PU"
  Divide2/1 -> fiften_PLUS_VB/1
  Constant2/1 -> Divide2/2
  Vb/1 -> Divide2/1  "Ta"
  Vc/1 -> Divide3/1  "Ta"
  Constant6/1 -> Divide3/2
  Divide3/1 -> fiften_PLUS_VC/1

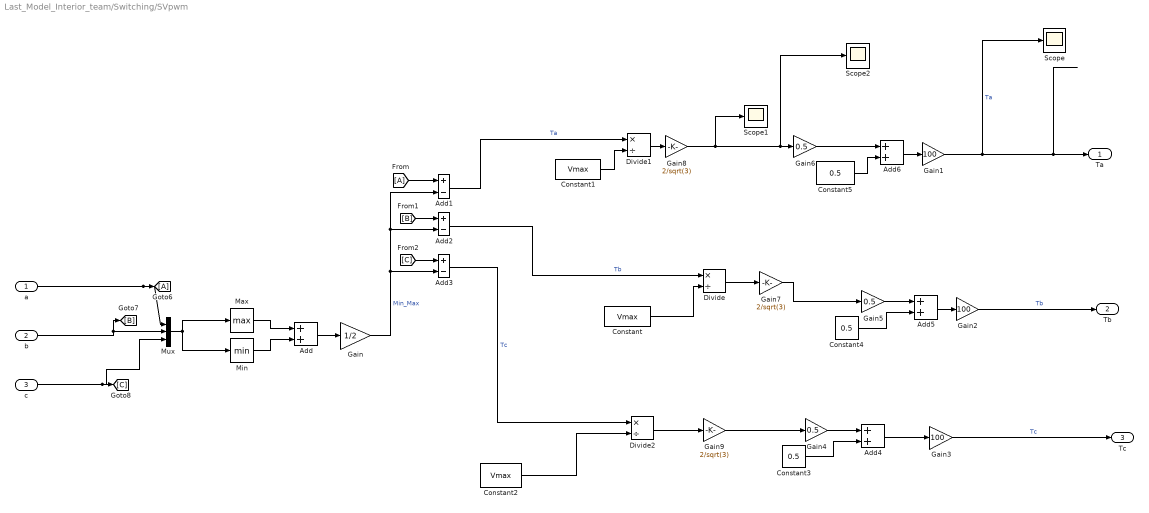
== system Last_Model_Interior_team/Switching/SVpwm ==
  a : Inport
  b : Inport  Port=2
  c : Inport  Port=3
  Add{,4..6} (4 alike) : Sum
  Add1 : Sum  Inputs=+-
  Add2 : Sum  Inputs=+-
  Add3 : Sum  Inputs=+-
  Constant : Constant  Value=Vmax
  Constant1 : Constant  Value=Vmax
  Constant2 : Constant  Value=Vmax
  Constant3 : Constant  Value=0.5
  Constant4 : Constant  Value=0.5
  Constant5 : Constant  Value=0.5
  Divide : Product  Inputs=*/
  Divide1 : Product  Inputs=*/
  Divide2 : Product  Inputs=*/
  Gain : Gain  Gain=1/2
  Gain1 : Gain  Gain=100
  Gain2 : Gain  Gain=100
  Gain3 : Gain  Gain=100
  Gain4 : Gain  Gain=0.5
  Gain5 : Gain  Gain=0.5
  Gain6 : Gain  Gain=0.5
  Gain7 : Gain  Gain=2/sqrt(3)
  Gain8 : Gain  Gain=2/sqrt(3)
  Gain9 : Gain  Gain=2/sqrt(3)
  Max : MinMax  Function=max
  Min : MinMax
  Mux : Mux  Inputs=3
  Scope : Scope
  Scope1 : Scope
  Scope2 : Scope
  Ta : Outport
  Tb : Outport  Port=2
  Tc : Outport  Port=3
  wires:
  c/1 -> Mux/3, [C]
  Add2/1 -> Divide/1  "Tb"
  [A] -> Add1/1
  a/1 -> [A], Mux/1
  Add6/1 -> Gain1/1
  Gain6/1 -> Add6/1
  [C] -> Add3/1
  Constant2/1 -> Divide2/2
  Add5/1 -> Gain2/1
  Constant/1 -> Divide/2
  Gain/1 -> Add3/2, Add2/2, Add1/2  "Min_Max"
  b/1 -> [B], Mux/2
  Constant1/1 -> Divide1/2
  Add1/1 -> Divide1/1  "Ta"
  Gain4/1 -> Add4/1
  Gain1/1 -> Ta/1, Scope/1  "Ta"
  Constant4/1 -> Add5/2
  Add/1 -> Gain/1
  Add3/1 -> Divide2/1  "Tc"
  Gain5/1 -> Add5/1
  Mux/1 -> Min/1, Max/1
  Constant3/1 -> Add4/2
  Min/1 -> Add/2
  Divide/1 -> Gain7/1
  Divide1/1 -> Gain8/1
  Gain2/1 -> Tb/1  "Tb"
  Gain3/1 -> Tc/1  "Tc"
  Divide2/1 -> Gain9/1
  Add4/1 -> Gain3/1
  Max/1 -> Add/1
  [B] -> Add2/1
  Constant5/1 -> Add6/2
  Gain9/1 -> Gain4/1
  Gain7/1 -> Gain5/1
  Gain8/1 -> Scope1/1, Scope2/1, Gain6/1

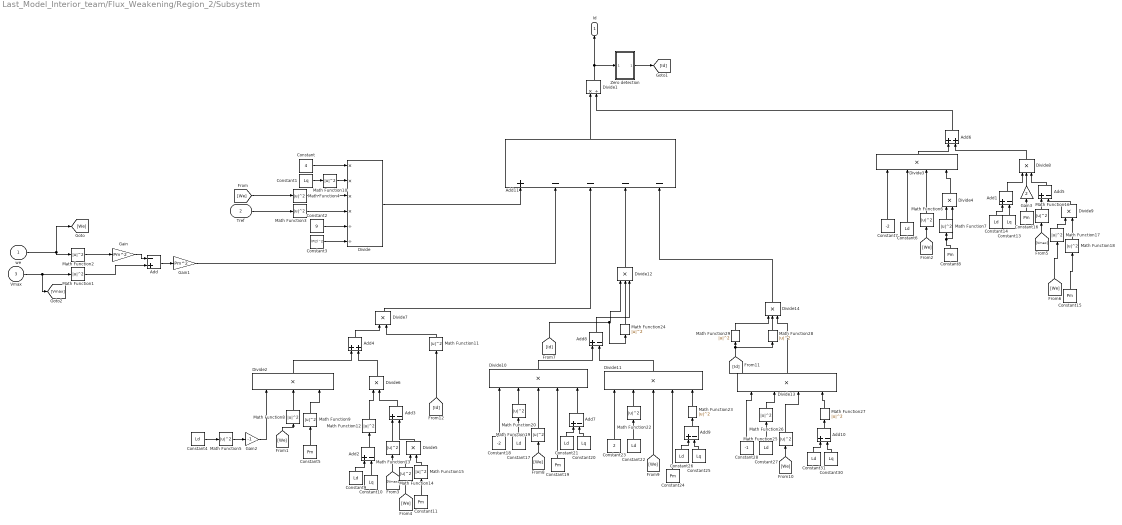
== system Last_Model_Interior_team/Flux_Weakening/Region_2/Subsystem ==
  we : Inport
  Tref : Inport  Port=2
  Vmax : Inport  Port=3
  Add : Sum  Inputs=-+
  Add{1..3,5,7..10} (8 alike) : Sum  Inputs=+-
  Add11 : Sum  Inputs=+----
  Add4 : Sum
  Add6 : Sum
  Constant : Constant  Value=4
  Constant{1,10,13,20,25,30} (6 alike) : Constant  Value=Lq
  Constant{5,8,11,15..16,19,24} (7 alike) : Constant  Value=Pm
  Constant{4,6,9,14,17,21..22,26..27,31} (10 alike) : Constant  Value=Ld
  Constant18 : Constant  Value=-2
  Constant2 : Constant  Value=9
  Constant23 : Constant  Value=2
  Constant28 : Constant  Value=-1
  Constant3 : Constant  Value=(P/2)^2
  Constant7 : Constant  Value=-2
  Divide : Product  Inputs=****//
  Divide1 : Product  Inputs=*/  RndMeth=Zero  SaturateOnIntegerOverflow=on
  Divide10 : Product  Inputs=*****  RndMeth=Zero  SaturateOnIntegerOverflow=on
  Divide11 : Product  Inputs=*****  RndMeth=Zero  SaturateOnIntegerOverflow=on
  Divide{2,8,12,14} (4 alike) : Product  Inputs=***  RndMeth=Zero  SaturateOnIntegerOverflow=on
  Divide13 : Product  Inputs=****  RndMeth=Zero  SaturateOnIntegerOverflow=on
  Divide3 : Product  Inputs=****  RndMeth=Zero  SaturateOnIntegerOverflow=on
  Divide4 : Product  Inputs=**
  Divide{5..7,9} (4 alike) : Product  Inputs=**  RndMeth=Zero  SaturateOnIntegerOverflow=on
  Gain : Gain  Gain=Pm^2
  Gain1 : Gain  Gain=Pm^2
  Gain2 : Gain  Gain=-1
  Gain3 : Gain  Gain=2
  Math Function{1..20,22..29} (28 alike) : Math  Operator=magnitude^2  OutputSignalType=real  SaturateOnIntegerOverflow=on
  Zero detection : Subsystem
  Id : Outport
  wires:
  Vmax/1 -> [Vmax], Math Function1/1
  Math Function1/1 -> Add/2
  we/1 -> [We], Math Function2/1
  Math Function2/1 -> Gain/1
  Gain/1 -> Add/1
  Tref/1 -> Math Function3/1
  Math Function3/1 -> Divide/4
  Constant/1 -> Divide/1
  Constant1/1 -> Math Function10/1
  [We] -> Math Function4/1
  Math Function4/1 -> Divide/3
  Constant2/1 -> Divide/5
  Constant3/1 -> Divide/6
  Constant4/1 -> Math Function5/1
  Math Function5/1 -> Gain2/1
  Gain2/1 -> Divide2/1
  [We] -> Math Function8/1
  Math Function8/1 -> Divide2/2
  Constant5/1 -> Math Function9/1
  Math Function9/1 -> Divide2/3
  Constant6/1 -> Divide3/2
  Constant7/1 -> Divide3/1
  [We] -> Math Function6/1
  Math Function6/1 -> Divide3/3
  Constant8/1 -> Divide4/2, Math Function7/1
  Math Function7/1 -> Divide4/1
  Math Function10/1 -> Divide/2
  Divide4/1 -> Divide3/4
  Add/1 -> Gain1/1
  Divide1/1 -> Zero detection/1(In1), Id/1
  [Id] -> Math Function11/1
  Math Function11/1 -> Divide7/2
  Constant9/1 -> Add2/1
  Constant10/1 -> Add2/2
  Add2/1 -> Math Function12/1
  [Vmax] -> Math Function13/1
  Math Function13/1 -> Add3/1
  [We] -> Math Function14/1
  Constant11/1 -> Math Function15/1
  Math Function14/1 -> Divide5/1
  Math Function15/1 -> Divide5/2
  Divide5/1 -> Add3/2
  Math Function12/1 -> Divide6/1
  Add3/1 -> Divide6/2
  Divide2/1 -> Add4/1
  Divide6/1 -> Add4/2
  Add4/1 -> Divide7/1
  Constant13/1 -> Add1/2
  Constant14/1 -> Add1/1
  Add1/1 -> Divide8/1
  [Vmax] -> Math Function16/1
  Math Function16/1 -> Add5/1
  [We] -> Math Function17/1
  Math Function17/1 -> Divide9/1
  Constant15/1 -> Math Function18/1
  Math Function18/1 -> Divide9/2
  Divide9/1 -> Add5/2
  Add5/1 -> Divide8/3
  Constant16/1 -> Gain3/1
  Gain3/1 -> Divide8/2
  Divide3/1 -> Add6/1
  Divide8/1 -> Add6/2
  Add6/1 -> Divide1/2
  Math Function19/1 -> Divide10/3
  [We] -> Math Function19/1
  Constant18/1 -> Divide10/1
  Constant17/1 -> Math Function20/1
  Constant19/1 -> Divide10/4
  Math Function20/1 -> Divide10/2
  Constant20/1 -> Add7/2
  Constant21/1 -> Add7/1
  Add7/1 -> Divide10/5
  Divide10/1 -> Add8/1
  Add9/1 -> Math Function23/1
  Constant26/1 -> Add9/1
  Constant25/1 -> Add9/2
  Math Function22/1 -> Divide11/2
  Constant24/1 -> Divide11/4
  Constant22/1 -> Math Function22/1
  Constant23/1 -> Divide11/1
  [We] -> Divide11/3
  Divide11/1 -> Add8/2
  Math Function23/1 -> Divide11/5
  [Id] -> Divide12/1, Math Function24/1
  Add8/1 -> Divide12/3
  Math Function24/1 -> Divide12/2
  Math Function25/1 -> Divide13/3
  [We] -> Math Function25/1
  Constant28/1 -> Divide13/1
  Constant27/1 -> Math Function26/1
  Math Function26/1 -> Divide13/2
  Constant30/1 -> Add10/2
  Constant31/1 -> Add10/1
  Add10/1 -> Math Function27/1
  Math Function28/1 -> Divide14/2
  [Id] -> Math Function29/1, Math Function28/1
  Math Function29/1 -> Divide14/1
  Divide13/1 -> Divide14/3
  Divide/1 -> Add11/1
  Gain1/1 -> Add11/2
  Divide7/1 -> Add11/3
  Divide12/1 -> Add11/4
  Divide14/1 -> Add11/5
  Add11/1 -> Divide1/1
  Math Function27/1 -> Divide13/4
  Zero detection/1(Out1) -> [Id]

== system Last_Model_Interior_team/Flux_Weakening/Region_3/Subsystem1 ==
  We : Inport
  Vmax : Inport  Port=2
  Abs : Abs
  Add : Sum
  Add1 : Sum  Inputs=+-
  Add2 : Sum  Inputs=++-
  Constant : Constant  Value=(Ld*Pm)/((Ld^2)-(Lq^2))
  Constant1 : Constant  Value=(Ld^2)*(Pm^2)
  Constant2 : Constant  Value=(Ld^2)-(Lq^2)
  Constant3 : Constant  Value=Pm^2
  Constant4 : Constant  Value=(Lq^2)*(Imax^2)
  Constant5 : Constant  Value=(Ld^2)-(Lq^2)
  Divide : Product  Inputs=**
  Divide1 : Product  Inputs=*/
  Divide2 : Product  Inputs=*/
  Square : Math  Operator=square  SaturateOnIntegerOverflow=on
  Square Root : Sqrt  SaturateOnIntegerOverflow=on
  Square1 : Math  Operator=square  SaturateOnIntegerOverflow=on
  Id : Outport
  wires:
  Constant/1 -> Add/1
  Constant1/1 -> Add1/1
  Constant2/1 -> Divide/1
  Constant3/1 -> Add2/1
  Constant4/1 -> Add2/2
  Vmax/1 -> Square/1
  We/1 -> Square1/1
  Square/1 -> Divide1/1
  Square1/1 -> Divide1/2
  Divide1/1 -> Add2/3
  Add2/1 -> Divide/2
  Divide/1 -> Add1/2
  Add1/1 -> Abs/1
  Square Root/1 -> Divide2/1
  Abs/1 -> Square Root/1
  Constant5/1 -> Divide2/2
  Divide2/1 -> Add/2
  Add/1 -> Id/1

== system Last_Model_Interior_team/Flux_Weakening/Saturation limits/Zero detection ==
  In1 : Inport
  Constant : Constant  Value=eps
  Switch : Switch  Criteria=u2 > Threshold  Threshold=eps
  Out1 : Outport
  wires:
  Switch/1 -> Out1/1
  Constant/1 -> Switch/3
  In1/1 -> Switch/2, Switch/1

== system Last_Model_Interior_team/Switching/+120_deg_Dpwm/Sector1 ==
  Vabc : Inport
  Enable : EnablePort
  Compare To Zero : simulink/Logic and Bit Operations/Compare To Zero  relop=<  OutDataTypeStr=boolean
  Compare To Zero1 : simulink/Logic and Bit Operations/Compare To Zero  relop=>=  OutDataTypeStr=boolean
  Demux : Demux  Outputs=3
  Enabled Subsystem : Subsystem  TreatAsAtomicUnit=on
  Enabled Subsystem1 : Subsystem  TreatAsAtomicUnit=on
  Merge : Merge
  Terminator : Terminator
  Terminator1 : Terminator
  Out1 : Outport
  wires:
  Demux/3 -> Terminator1/1
  Demux/2 -> Terminator/1
  Demux/1 -> Compare To Zero/1, Compare To Zero1/1
  Vabc/1 -> Demux/1, Enabled Subsystem1/1(Vabc), Enabled Subsystem/1(Vabc)
  Merge/1 -> Out1/1
  Enabled Subsystem1/1(Out1) -> Merge/2
  Enabled Subsystem/1(Out1) -> Merge/1
  Compare To Zero1/1 -> Enabled Subsystem1/Enable
  Compare To Zero/1 -> Enabled Subsystem/Enable

== system Last_Model_Interior_team/Switching/+120_deg_Dpwm/Sector2 ==
  Vabc : Inport
  Enable : EnablePort
  Compare To Zero : simulink/Logic and Bit Operations/Compare To Zero  relop=<  OutDataTypeStr=boolean
  Compare To Zero1 : simulink/Logic and Bit Operations/Compare To Zero  relop=>=  OutDataTypeStr=boolean
  Demux : Demux  Outputs=3
  Enabled Subsystem : Subsystem  TreatAsAtomicUnit=on
  Enabled Subsystem1 : Subsystem  TreatAsAtomicUnit=on
  Merge : Merge
  Terminator : Terminator
  Terminator1 : Terminator
  Out1 : Outport
  wires:
  Demux/1 -> Terminator/1
  Compare To Zero/1 -> Enabled Subsystem/Enable
  Compare To Zero1/1 -> Enabled Subsystem1/Enable
  Enabled Subsystem/1(Out1) -> Merge/1
  Enabled Subsystem1/1(Out1) -> Merge/2
  Merge/1 -> Out1/1
  Vabc/1 -> Enabled Subsystem1/1(Vabc), Enabled Subsystem/1(Vabc), Demux/1
  Demux/3 -> Compare To Zero1/1, Compare To Zero/1
  Demux/2 -> Terminator1/1

== system Last_Model_Interior_team/Switching/+120_deg_Dpwm/Sector3 ==
  Vabc : Inport
  Enable : EnablePort
  Compare To Zero : simulink/Logic and Bit Operations/Compare To Zero  relop=<  OutDataTypeStr=boolean
  Compare To Zero1 : simulink/Logic and Bit Operations/Compare To Zero  relop=>=  OutDataTypeStr=boolean
  Demux : Demux  Outputs=3
  Enabled Subsystem : Subsystem  TreatAsAtomicUnit=on
  Enabled Subsystem1 : Subsystem  TreatAsAtomicUnit=on
  Merge : Merge
  Terminator : Terminator
  Terminator1 : Terminator
  Out1 : Outport
  wires:
  Demux/2 -> Terminator1/1
  Demux/3 -> Compare To Zero/1, Compare To Zero1/1
  Vabc/1 -> Demux/1, Enabled Subsystem/1(Vabc), Enabled Subsystem1/1(Vabc)
  Merge/1 -> Out1/1
  Enabled Subsystem1/1(Out1) -> Merge/2
  Enabled Subsystem/1(Out1) -> Merge/1
  Compare To Zero1/1 -> Enabled Subsystem1/Enable
  Compare To Zero/1 -> Enabled Subsystem/Enable
  Demux/1 -> Terminator/1

== system Last_Model_Interior_team/Switching/+120_deg_Dpwm/Sector4 ==
  Vabc : Inport
  Enable : EnablePort
  Compare To Zero : simulink/Logic and Bit Operations/Compare To Zero  relop=<  OutDataTypeStr=boolean
  Compare To Zero1 : simulink/Logic and Bit Operations/Compare To Zero  relop=>=  OutDataTypeStr=boolean
  Demux : Demux  Outputs=3
  Enabled Subsystem : Subsystem  TreatAsAtomicUnit=on
  Enabled Subsystem1 : Subsystem  TreatAsAtomicUnit=on
  Merge : Merge
  Terminator : Terminator
  Terminator1 : Terminator
  Out1 : Outport
  wires:
  Demux/3 -> Terminator/1
  Demux/1 -> Compare To Zero/1, Compare To Zero1/1
  Compare To Zero/1 -> Enabled Subsystem/Enable
  Compare To Zero1/1 -> Enabled Subsystem1/Enable
  Enabled Subsystem/1(Out1) -> Merge/1
  Enabled Subsystem1/1(Out1) -> Merge/2
  Merge/1 -> Out1/1
  Vabc/1 -> Enabled Subsystem/1(Vabc), Enabled Subsystem1/1(Vabc), Demux/1
  Demux/2 -> Terminator1/1

== system Last_Model_Interior_team/Switching/+120_deg_Dpwm/Sector5 ==
  Vabc : Inport
  Enable : EnablePort
  Compare To Zero : simulink/Logic and Bit Operations/Compare To Zero  relop=<  OutDataTypeStr=boolean
  Compare To Zero1 : simulink/Logic and Bit Operations/Compare To Zero  relop=>=  OutDataTypeStr=boolean
  Demux : Demux  Outputs=3
  Enabled Subsystem : Subsystem  TreatAsAtomicUnit=on
  Enabled Subsystem1 : Subsystem  TreatAsAtomicUnit=on
  Merge : Merge
  Terminator : Terminator
  Terminator1 : Terminator
  Out1 : Outport
  wires:
  Demux/1 -> Terminator1/1
  Demux/2 -> Compare To Zero1/1, Compare To Zero/1
  Vabc/1 -> Demux/1, Enabled Subsystem1/1(Vabc), Enabled Subsystem/1(Vabc)
  Merge/1 -> Out1/1
  Enabled Subsystem1/1(Out1) -> Merge/2
  Enabled Subsystem/1(Out1) -> Merge/1
  Compare To Zero1/1 -> Enabled Subsystem1/Enable
  Compare To Zero/1 -> Enabled Subsystem/Enable
  Demux/3 -> Terminator/1

== system Last_Model_Interior_team/Switching/+120_deg_Dpwm/Sector6 ==
  Vabc : Inport
  Enable : EnablePort
  Compare To Zero : simulink/Logic and Bit Operations/Compare To Zero  relop=<  OutDataTypeStr=boolean
  Compare To Zero1 : simulink/Logic and Bit Operations/Compare To Zero  relop=>=  OutDataTypeStr=boolean
  Demux : Demux  Outputs=3
  Enabled Subsystem : Subsystem  TreatAsAtomicUnit=on
  Enabled Subsystem1 : Subsystem  TreatAsAtomicUnit=on
  Merge : Merge
  Terminator : Terminator
  Terminator1 : Terminator
  Out1 : Outport
  wires:
  Demux/2 -> Terminator/1
  Demux/3 -> Compare To Zero/1, Compare To Zero1/1
  Compare To Zero/1 -> Enabled Subsystem/Enable
  Compare To Zero1/1 -> Enabled Subsystem1/Enable
  Enabled Subsystem/1(Out1) -> Merge/1
  Enabled Subsystem1/1(Out1) -> Merge/2
  Merge/1 -> Out1/1
  Vabc/1 -> Enabled Subsystem/1(Vabc), Enabled Subsystem1/1(Vabc), Demux/1
  Demux/1 -> Terminator1/1

== system Last_Model_Interior_team/Switching/-120_deg_Dpwm/Sector1 ==
  Vabc : Inport
  Enable : EnablePort
  Compare To Zero : simulink/Logic and Bit Operations/Compare To Zero  relop=<  OutDataTypeStr=boolean
  Compare To Zero1 : simulink/Logic and Bit Operations/Compare To Zero  relop=>=  OutDataTypeStr=boolean
  Demux : Demux  Outputs=3
  Enabled Subsystem : Subsystem  TreatAsAtomicUnit=on
  Enabled Subsystem1 : Subsystem  TreatAsAtomicUnit=on
  Merge : Merge
  Terminator : Terminator
  Terminator1 : Terminator
  Out1 : Outport
  wires:
  Compare To Zero/1 -> Enabled Subsystem/Enable
  Compare To Zero1/1 -> Enabled Subsystem1/Enable
  Enabled Subsystem/1(Out1) -> Merge/1
  Enabled Subsystem1/1(Out1) -> Merge/2
  Merge/1 -> Out1/1
  Vabc/1 -> Enabled Subsystem/1(Vabc), Enabled Subsystem1/1(Vabc), Demux/1
  Demux/1 -> Compare To Zero1/1, Compare To Zero/1
  Demux/2 -> Terminator/1
  Demux/3 -> Terminator1/1

== system Last_Model_Interior_team/Switching/-120_deg_Dpwm/Sector2 ==
  Vabc : Inport
  Enable : EnablePort
  Compare To Zero : simulink/Logic and Bit Operations/Compare To Zero  relop=<  OutDataTypeStr=boolean
  Compare To Zero1 : simulink/Logic and Bit Operations/Compare To Zero  relop=>=  OutDataTypeStr=boolean
  Demux : Demux  Outputs=3
  Enabled Subsystem : Subsystem  TreatAsAtomicUnit=on
  Enabled Subsystem1 : Subsystem  TreatAsAtomicUnit=on
  Merge : Merge
  Terminator : Terminator
  Terminator1 : Terminator
  Out1 : Outport
  wires:
  Demux/2 -> Terminator1/1
  Demux/3 -> Compare To Zero/1, Compare To Zero1/1
  Vabc/1 -> Demux/1, Enabled Subsystem/1(Vabc), Enabled Subsystem1/1(Vabc)
  Merge/1 -> Out1/1
  Enabled Subsystem1/1(Out1) -> Merge/2
  Enabled Subsystem/1(Out1) -> Merge/1
  Compare To Zero1/1 -> Enabled Subsystem1/Enable
  Compare To Zero/1 -> Enabled Subsystem/Enable
  Demux/1 -> Terminator/1

== system Last_Model_Interior_team/Switching/-120_deg_Dpwm/Sector3 ==
  Vabc : Inport
  Enable : EnablePort
  Compare To Zero : simulink/Logic and Bit Operations/Compare To Zero  relop=<  OutDataTypeStr=boolean
  Compare To Zero1 : simulink/Logic and Bit Operations/Compare To Zero  relop=>=  OutDataTypeStr=boolean
  Demux : Demux  Outputs=3
  Enabled Subsystem : Subsystem  TreatAsAtomicUnit=on
  Enabled Subsystem1 : Subsystem  TreatAsAtomicUnit=on
  Merge : Merge
  Terminator : Terminator
  Terminator1 : Terminator
  Out1 : Outport
  wires:
  Demux/1 -> Terminator/1
  Compare To Zero/1 -> Enabled Subsystem/Enable
  Compare To Zero1/1 -> Enabled Subsystem1/Enable
  Enabled Subsystem/1(Out1) -> Merge/1
  Enabled Subsystem1/1(Out1) -> Merge/2
  Merge/1 -> Out1/1
  Vabc/1 -> Enabled Subsystem1/1(Vabc), Enabled Subsystem/1(Vabc), Demux/1
  Demux/3 -> Compare To Zero1/1, Compare To Zero/1
  Demux/2 -> Terminator1/1

== system Last_Model_Interior_team/Switching/-120_deg_Dpwm/Sector4 ==
  Vabc : Inport
  Enable : EnablePort
  Compare To Zero : simulink/Logic and Bit Operations/Compare To Zero  relop=<  OutDataTypeStr=boolean
  Compare To Zero1 : simulink/Logic and Bit Operations/Compare To Zero  relop=>=  OutDataTypeStr=boolean
  Demux : Demux  Outputs=3
  Enabled Subsystem : Subsystem  TreatAsAtomicUnit=on
  Enabled Subsystem1 : Subsystem  TreatAsAtomicUnit=on
  Merge : Merge
  Terminator : Terminator
  Terminator1 : Terminator
  Out1 : Outport
  wires:
  Demux/2 -> Terminator1/1
  Vabc/1 -> Demux/1, Enabled Subsystem1/1(Vabc), Enabled Subsystem/1(Vabc)
  Merge/1 -> Out1/1
  Enabled Subsystem1/1(Out1) -> Merge/2
  Enabled Subsystem/1(Out1) -> Merge/1
  Compare To Zero1/1 -> Enabled Subsystem1/Enable
  Compare To Zero/1 -> Enabled Subsystem/Enable
  Demux/1 -> Compare To Zero1/1, Compare To Zero/1
  Demux/3 -> Terminator/1

== system Last_Model_Interior_team/Switching/-120_deg_Dpwm/Sector5 ==
  Vabc : Inport
  Enable : EnablePort
  Compare To Zero : simulink/Logic and Bit Operations/Compare To Zero  relop=<  OutDataTypeStr=boolean
  Compare To Zero1 : simulink/Logic and Bit Operations/Compare To Zero  relop=>=  OutDataTypeStr=boolean
  Demux : Demux  Outputs=3
  Enabled Subsystem : Subsystem  TreatAsAtomicUnit=on
  Enabled Subsystem1 : Subsystem  TreatAsAtomicUnit=on
  Merge : Merge
  Terminator : Terminator
  Terminator1 : Terminator
  Out1 : Outport
  wires:
  Demux/3 -> Terminator/1
  Compare To Zero/1 -> Enabled Subsystem/Enable
  Compare To Zero1/1 -> Enabled Subsystem1/Enable
  Enabled Subsystem/1(Out1) -> Merge/1
  Enabled Subsystem1/1(Out1) -> Merge/2
  Merge/1 -> Out1/1
  Vabc/1 -> Enabled Subsystem/1(Vabc), Enabled Subsystem1/1(Vabc), Demux/1
  Demux/2 -> Compare To Zero/1, Compare To Zero1/1
  Demux/1 -> Terminator1/1

== system Last_Model_Interior_team/Switching/-120_deg_Dpwm/Sector6 ==
  Vabc : Inport
  Enable : EnablePort
  Compare To Zero : simulink/Logic and Bit Operations/Compare To Zero  relop=<  OutDataTypeStr=boolean
  Compare To Zero1 : simulink/Logic and Bit Operations/Compare To Zero  relop=>=  OutDataTypeStr=boolean
  Demux : Demux  Outputs=3
  Enabled Subsystem : Subsystem  TreatAsAtomicUnit=on
  Enabled Subsystem1 : Subsystem  TreatAsAtomicUnit=on
  Merge : Merge
  Terminator : Terminator
  Terminator1 : Terminator
  Out1 : Outport
  wires:
  Demux/1 -> Terminator1/1
  Demux/2 -> Compare To Zero1/1, Compare To Zero/1
  Vabc/1 -> Demux/1, Enabled Subsystem1/1(Vabc), Enabled Subsystem/1(Vabc)
  Merge/1 -> Out1/1
  Enabled Subsystem1/1(Out1) -> Merge/2
  Enabled Subsystem/1(Out1) -> Merge/1
  Compare To Zero1/1 -> Enabled Subsystem1/Enable
  Compare To Zero/1 -> Enabled Subsystem/Enable
  Demux/3 -> Terminator/1

== system Last_Model_Interior_team/Switching/30_deg_Dpwm/Sector1 ==
  Vabc : Inport
  Enable : EnablePort
  Compare To Zero : simulink/Logic and Bit Operations/Compare To Zero  relop=<  OutDataTypeStr=boolean
  Compare To Zero1 : simulink/Logic and Bit Operations/Compare To Zero  relop=>=  OutDataTypeStr=boolean
  Demux : Demux  Outputs=3
  Enabled Subsystem : Subsystem  TreatAsAtomicUnit=on
  Enabled Subsystem1 : Subsystem  TreatAsAtomicUnit=on
  Merge : Merge
  Terminator : Terminator
  Terminator1 : Terminator
  Out1 : Outport
  wires:
  Demux/3 -> Terminator1/1
  Demux/2 -> Terminator/1
  Demux/1 -> Compare To Zero/1, Compare To Zero1/1
  Vabc/1 -> Demux/1, Enabled Subsystem1/1(Vabc), Enabled Subsystem/1(Vabc)
  Merge/1 -> Out1/1
  Enabled Subsystem1/1(Out1) -> Merge/2
  Enabled Subsystem/1(Out1) -> Merge/1
  Compare To Zero1/1 -> Enabled Subsystem1/Enable
  Compare To Zero/1 -> Enabled Subsystem/Enable
